simulink model "GeneralFramework"  (R2022a)
settings: Solver=ode23tb  StartTime=0.0  StopTime=t_sim  RelTol=1e-3
values from neighbouring files (symbols this model uses):
  AccPwrbp = [0 3.0779560993538198]    [Init_Parameters.m]
  AccSpdbp = [256.49641719585139 641.24104298962845]    [Init_Parameters.m]
  EngTrqSat = 60    [Init_Parameters.m]
  f_mu = ones(4,1)    [Init_Parameters.m]
  InitialLatPosition = 0    [Init_Parameters.m]
  numWheels = 4    [Init_Parameters.m]    (also in VehicleParameters.m)
  omega_hw = 13.51    [Init_Parameters.m]
  steerDir = -1    [Init_Parameters.m]
  t_start = 1    [Init_Parameters.m]
  t_stop = 100    [Init_Parameters.m]
  theta_max = 270    [Init_Parameters.m]
  TrackWidth = VEH.TrackWidth    [Init_Parameters.m]
  Trans = data.Trans    [Init_Parameters.m]    (also in ModelWorkspace.mat = )
  VEH = data.VEH    [Init_Parameters.m]    (also in ModelWorkspace.mat = ; VehicleParameters.m)
  wheelB = VEH.FrontAxlePositionfromCG+VEH.RearAxlePositionfromCG    [Init_Parameters.m]    (also in VehicleParameters.m)
  xdot_r = 2    [Init_Parameters.m]
libraries: autolibutils x10, simulink x8, sharedtransform x5, autolibsharedcoupling x3, vehdynlibsuspension x2, shared6dof x2, autolibtranscontrolscommon x1, vehdynlibdriver x1, autolibsharedtransfixedgear x1, vehdynlibsteering x1, autolibshareddiff x1, autolibsharedmappedengines x1
(part 3 of 5)

== system GeneralFramework/Passanger Vehicle/Pedal Cluster Input ==
  Driver : Inport
  Driveline : Inport  Port=2
  Steering : Inport  Port=3
  Bus Selector : BusSelector  OutputSignals=SteerCmd,AccelCmd,DecelCmd,GearCmd
  Bus Selector1 : BusSelector  OutputSignals=BrkPrs
  Bus Selector2 : BusSelector  OutputSignals=StrWhlTrq
  SteerCmd : Outport  VectorParamsAs1DForOutWhenUnconnected=off
  AccelCmd : Outport  Port=2  VectorParamsAs1DForOutWhenUnconnected=off
  DecelCmd : Outport  Port=3  VectorParamsAs1DForOutWhenUnconnected=off
  GearCmd : Outport  Port=4  VectorParamsAs1DForOutWhenUnconnected=off
  BrkPrs : Outport  Port=5  VectorParamsAs1DForOutWhenUnconnected=off
  StrWhlTrq : Outport  Port=6  VectorParamsAs1DForOutWhenUnconnected=off
  wires:
  Bus Selector/2 -> AccelCmd/1  "<AccelCmd>"
  Driver/1 -> Bus Selector/1
  Bus Selector/3 -> DecelCmd/1  "<DecelCmd>"
  Bus Selector/4 -> GearCmd/1  "<GearCmd>"
  Bus Selector/1 -> SteerCmd/1  "<SteerCmd>"
  Driveline/1 -> Bus Selector1/1
  Bus Selector1/1 -> BrkPrs/1  "<BrkPrs>"
  Steering/1 -> Bus Selector2/1
  Bus Selector2/1 -> StrWhlTrq/1  "<StrWhlTrq>"

== system GeneralFramework/Passanger Vehicle/Pedal Cluster Output ==
  SteerFdbk : Inport
  AccFdbk : Inport  Port=2
  DecelFdbk : Inport  Port=3
  GearFdbk : Inport  Port=4
  Bus Creator1 : BusCreator  Inputs=4
  Signal Specification : SignalSpecification  Unit=rad
  Signal Specification1 : SignalSpecification  Unit=1
  Signal Specification2 : SignalSpecification  Unit=1
  Signal Specification3 : SignalSpecification  Unit=1
  OperatorFdbk : Outport
  wires:
  Signal Specification1/1 -> Bus Creator1/2  "AccFdbk"
  Signal Specification3/1 -> Bus Creator1/4  "GearFdbk"
  AccFdbk/1 -> Signal Specification1/1
  DecelFdbk/1 -> Signal Specification2/1
  GearFdbk/1 -> Signal Specification3/1
  Signal Specification/1 -> Bus Creator1/1  "SteerFdbk"
  SteerFdbk/1 -> Signal Specification/1
  Bus Creator1/1 -> OperatorFdbk/1
  Signal Specification2/1 -> Bus Creator1/3  "DecelFdbk"

== system GeneralFramework/Passanger Vehicle/Pedal Cluster and cabin ==
  SteerCmd : Inport
  AccCmd : Inport  Port=2
  DecelCmd : Inport  Port=3
  GearCmd : Inport  Port=4
  BrkPrs : Inport  Port=5
  StrWhlTrq : Inport  Port=6
  Brake Pedal : Subsystem
  Dead Zone2 : DeadZone  LowerValue=0  UpperValue=.01  ZeroCross=off
  Dead Zone3 : DeadZone  LowerValue=-.01  UpperValue=.01  ZeroCross=off
  Terminator : Terminator
  Terminator1 : Terminator
  SteerFdbk : Outport
  AccFdbk : Outport  Port=2
  DecelFdbk : Outport  Port=3
  GearFdbk : Outport  Port=4
  wires:
  AccCmd/1 -> Dead Zone2/1
  GearCmd/1 -> GearFdbk/1
  Brake Pedal/1(DecelFdbk) -> DecelFdbk/1
  Dead Zone3/1 -> SteerFdbk/1
  StrWhlTrq/1 -> Terminator1/1
  DecelCmd/1 -> Brake Pedal/1(DecelCmd)
  SteerCmd/1 -> Dead Zone3/1
  BrkPrs/1 -> Terminator/1
  Dead Zone2/1 -> AccFdbk/1

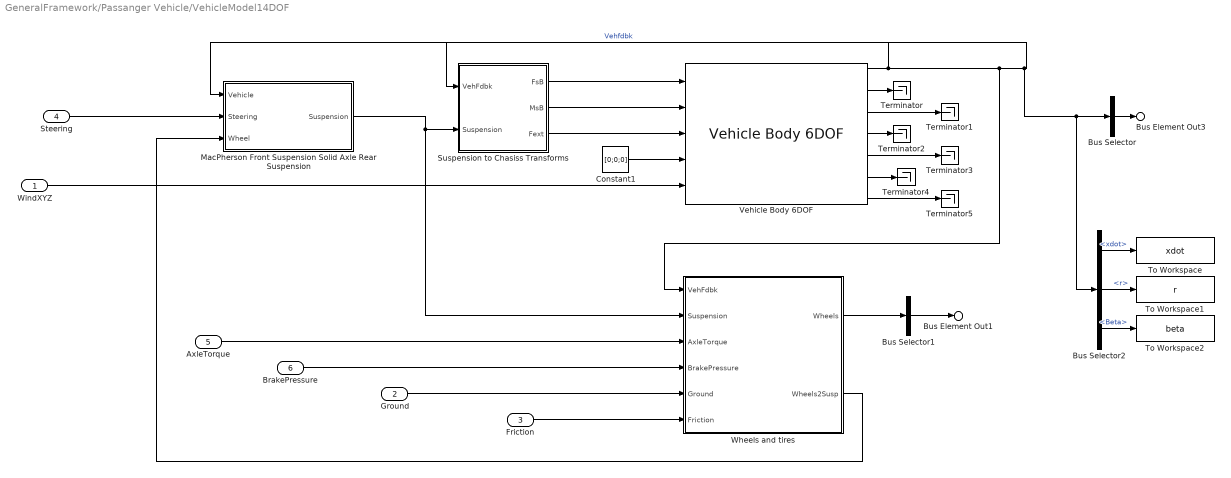
== system GeneralFramework/Passanger Vehicle/VehicleModel14DOF ==
  WindXYZ : Inport
  Ground : Inport  Port=2
  Friction : Inport  Port=3
  Steering : Inport  Port=4
  AxleTorque : Inport  Port=5
  BrakePressure : Inport  Port=6
  Bus Selector : BusSelector  OutputSignals=InertFrm,BdyFrm  OutputAsBus=on
  Bus Selector1 : BusSelector  OutputSignals=TireFrame,Steering  OutputAsBus=on
  Bus Selector2 : BusSelector  OutputSignals=BdyFrm.Cg.Vel.xdot,BdyFrm.Cg.AngVel.r,BdyFrm.Geom.Ang.Beta
  Constant1 : Constant  Value=[0;0;0]
  MacPherson Front Suspension Solid Axle Rear Suspension : Subsystem
  Suspension to Chasiss Transforms : Subsystem
  Terminator{,1..5} (6 alike) : Terminator
  To Workspace : ToWorkspace  VariableName=xdot  SampleTime=-1
      settings: Save2DSignal=2-D array (concatenate along first dimension)
  To Workspace1 : ToWorkspace  VariableName=r  SampleTime=-1
      settings: Save2DSignal=2-D array (concatenate along first dimension)
  To Workspace2 : ToWorkspace  VariableName=beta  SampleTime=-1
      settings: Save2DSignal=2-D array (concatenate along first dimension)
  Vehicle Body 6DOF : vehdynlibeom/Vehicle Body 6DOF  extPos=on  extVel=on  extEuler=on  extRotRate=on  htchFMode=off  htchMMode=off  m=VEH.Mass  a=VEH.FrontAxlePositionfromCG  b=VEH.RearAxlePositionfromCG  d=0  h=VEH.HeightCG  dh=1  hl=0  hh=0.1  Xe_o=[VEH.InitialLongPosition,InitialLatPosition,VEH.InitialVertPosition]  xbdot_o=[VEH.InitialLongVel,VEH.InitialLatVel,VEH.InitialVertVel]  eul_o=[VEH.InitialRollAngle,VEH.InitialPitchAngle,VEH.InitialYawAngle]  p_o=[VEH.InitialRollRate,VEH.InitialPitchRate,VEH.InitialYawRate]  Iveh=[VEH.RollMomentInertia 0 0; 0 VEH.PitchMomentInertia 0; 0 0 VEH.YawMomentInertia]  w=VEH.TrackWidth.*[1 1]  z1m=0  z1R=[-.25,.125,.15]  z1I=[1.4,-.2,.1;-.2,1.4,.1;.1,.1,2.25].*0  z2m=0  z2R=[1.4,0,.8]  z2I=[1.4,-.2,.1;-.2,1.4,.1;.1,.1,2.25].*0  z3m=0  z3R=[.75,-.5,.4]  z3I=[5,-.1,-2;-2,9,.1;-.1,.1,6].*0  z4m=0  z4R=[.75,.5,.4]  z4I=[5,-.1,-2;-2,9,.1;-.1,.1,6].*0  z5m=0  z5R=[1.25,-.5,.4]  z5I=[5,-.1,-2;-2,9,.1;-.1,.1,6].*0  z6m=0  z6R=[1.25,-.5,.4]  z6I=[5,-.1,-2;-2,9,.1;-.1,.1,6].*0  z7m=0  z7R=[2,0,.25]  z7I=[1.4,-.2,.1;-.2,1.4,.1;.1,.1,2.25].*0  Af=VEH.FrontalArea  Cd=.3  Cl=.1  Cpm=.1  beta_w=[0 0.01:0.01:0.3]  Cs=[0 0.01:0.01:0.3]  Cym=[0 1e-6:0.01:0.3]  Pabs=101325  extTamb=off  Tair=273  g=9.81  xdot_tol=.1  longOff=0  latOff=0  vertOff=0.0112  wrapAng=off  aMode=2
      settings: SourceProductBaseCode=VE
  Wheels and tires : Subsystem
  Bus Element Out3 : Outport  PortName=Vehfdbk
  Bus Element Out1 : Outport  Port=2  PortName=Wheels
  wires:
  Ground/1 -> Wheels and tires/5(Ground)
  MacPherson Front Suspension Solid Axle Rear Suspension/1(Suspension) -> Wheels and tires/2(Suspension), Suspension to Chasiss Transforms/2(Suspension)
  Vehicle Body 6DOF/3 -> Terminator1/1
  Suspension to Chasiss Transforms/3(Fext) -> Vehicle Body 6DOF/3
  Vehicle Body 6DOF/7 -> Terminator5/1
  BrakePressure/1 -> Wheels and tires/4(BrakePressure)
  AxleTorque/1 -> Wheels and tires/3(AxleTorque)
  Vehicle Body 6DOF/6 -> Terminator4/1
  Vehicle Body 6DOF/5 -> Terminator3/1
  Constant1/1 -> Vehicle Body 6DOF/4
  Wheels and tires/2(Wheels2Susp) -> MacPherson Front Suspension Solid Axle Rear Suspension/3(Wheel)
  Vehicle Body 6DOF/4 -> Terminator2/1
  Suspension to Chasiss Transforms/1(FsB) -> Vehicle Body 6DOF/1
  Vehicle Body 6DOF/2 -> Terminator/1
  Suspension to Chasiss Transforms/2(MsB) -> Vehicle Body 6DOF/2
  WindXYZ/1 -> Vehicle Body 6DOF/5
  Steering/1 -> MacPherson Front Suspension Solid Axle Rear Suspension/2(Steering)
  Friction/1 -> Wheels and tires/6(Friction)
  Wheels and tires/1(Wheels) -> Bus Selector1/1
  Bus Selector1/1 -> Bus Element Out1/1
  Bus Selector/1 -> Bus Element Out3/1
  Vehicle Body 6DOF/1 -> Wheels and tires/1(VehFdbk), Bus Selector/1, Bus Selector2/1, MacPherson Front Suspension Solid Axle Rear Suspension/1(Vehicle), Suspension to Chasiss Transforms/1(VehFdbk)  "Vehfdbk"
  Bus Selector2/1 -> To Workspace/1  "<xdot>"
  Bus Selector2/2 -> To Workspace1/1  "<r>"
  Bus Selector2/3 -> To Workspace2/1  "<Beta>"

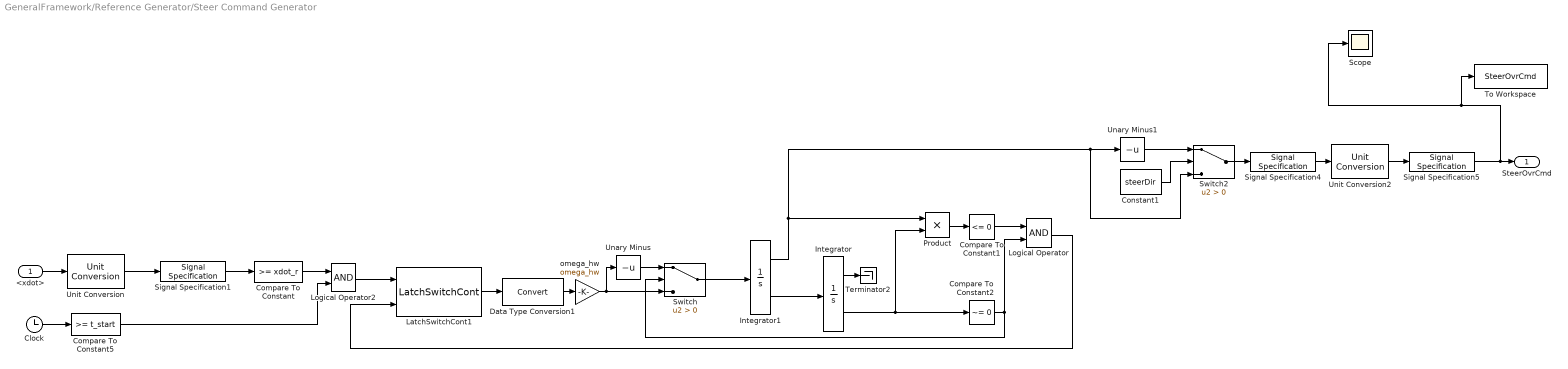
== system GeneralFramework/Reference Generator/Steer Command Generator ==
  <xdot> : Inport
  Clock : Clock
  Compare To Constant : simulink/Logic and Bit Operations/Compare To Constant  relop=>=  const=xdot_r  OutDataTypeStr=boolean
  Compare To Constant1 : simulink/Logic and Bit Operations/Compare To Constant  relop=<=  const=0  OutDataTypeStr=boolean
  Compare To Constant2 : simulink/Logic and Bit Operations/Compare To Constant  relop=~=  const=0  OutDataTypeStr=boolean  ZeroCross=off
  Compare To Constant5 : simulink/Logic and Bit Operations/Compare To Constant  relop=>=  const=t_start  OutDataTypeStr=boolean
  Constant1 : Constant  Value=steerDir
  Data Type Conversion1 : DataTypeConversion  SaturateOnIntegerOverflow=off  RndMeth=Floor
  Integrator : Integrator  LimitOutput=on  UpperSaturationLimit=t_stop  ShowSaturationPort=on
  Integrator1 : Integrator  LimitOutput=on  UpperSaturationLimit=theta_max  LowerSaturationLimit=-theta_max  ShowSaturationPort=on
  LatchSwitchCont1 : autolibutils/LatchSwitchCont  aMode=aMode
      settings: SourceProductBaseCode=PW,DR,MT,VE
  Logical Operator : Logic  AllPortsSameDT=off  OutDataTypeStr=boolean
  Logical Operator2 : Logic  AllPortsSameDT=off  OutDataTypeStr=boolean
  Product : Product
  Scope : Scope
  Signal Specification1 : SignalSpecification  Unit=mph
  Signal Specification4 : SignalSpecification  Unit=deg
  Signal Specification5 : SignalSpecification  Unit=rad
  Switch : Switch  Criteria=u2 > Threshold  SaturateOnIntegerOverflow=off  InputSameDT=off
  Switch2 : Switch  Criteria=u2 > Threshold  SaturateOnIntegerOverflow=off  InputSameDT=off
  Terminator2 : Terminator
  To Workspace : ToWorkspace  VariableName=SteerOvrCmd  SampleTime=-1
      settings: Save2DSignal=2-D array (concatenate along first dimension)
  Unary Minus : UnaryMinus
  Unary Minus1 : UnaryMinus
  Unit Conversion : UnitConversion
  Unit Conversion2 : UnitConversion
  omega_hw : Gain  Gain=omega_hw
  SteerOvrCmd : Outport  VectorParamsAs1DForOutWhenUnconnected=off
  wires:
  Unit Conversion2/1 -> Signal Specification5/1
  Unary Minus/1 -> Switch/1
  Compare To Constant/1 -> Logical Operator2/1
  Unary Minus1/1 -> Switch2/1
  Switch/1 -> Integrator1/1
  Signal Specification4/1 -> Unit Conversion2/1
  Integrator1/1 -> Product/1, Unary Minus1/1, Switch2/3
  omega_hw/1 -> Switch/3, Unary Minus/1
  Compare To Constant1/1 -> Logical Operator/1
  <xdot>/1 -> Unit Conversion/1
  Clock/1 -> Compare To Constant5/1
  Data Type Conversion1/1 -> omega_hw/1
  Product/1 -> Compare To Constant1/1
  Unit Conversion/1 -> Signal Specification1/1
  Integrator/2 -> Product/2, Compare To Constant2/1
  Switch2/1 -> Signal Specification4/1
  Integrator/1 -> Terminator2/1
  Compare To Constant5/1 -> Logical Operator2/2
  Compare To Constant2/1 -> Logical Operator/2, Switch/2
  Signal Specification1/1 -> Compare To Constant/1
  Logical Operator2/1 -> LatchSwitchCont1/1
  Integrator1/2 -> Integrator/1
  Logical Operator/1 -> LatchSwitchCont1/2
  Constant1/1 -> Switch2/2
  LatchSwitchCont1/1 -> Data Type Conversion1/1
  Signal Specification5/1 -> To Workspace/1, Scope/1, SteerOvrCmd/1

== system GeneralFramework/Visualization/3D Engine ==
  note: 1) Add Subsystem or Model blocks as valid variant choices.
      | 2) You cannot connect blocks at this level. At simulation, connectivity is automatically
      | determined, based on the active variant and port name matching.
  VehFdbk : Inport
  3D Engine : Subsystem  VariantControl=engine3D==1
  3D Engine Disabled : Subsystem  VariantControl=engine3D==2

== system GeneralFramework/Visualization/ISO 15037-1:2006 ==
  VehFdbk : Inport
  Disabled : Subsystem  VariantControl=0
  Enabled : Subsystem  VariantControl=1

== system GeneralFramework/Passanger Vehicle/Driveline Idea Fixed Gear/Brake Hydraulics ==
  BrkPrsCmd : Inport
  Circuit : Switch  Criteria=u2 ~= 0  SaturateOnIntegerOverflow=off  InputSameDT=off
  Constant : Constant  Value=-1
  Front Bias : Constant
  Gain4 : Gain  Gain=8e6
  Mux : Mux
  Product : Product
  Rear Bias : Constant  Value=.6
  Scope : Scope
  Spool : Gain  Gain=50
  Subtract : Sum  Inputs=+-
  Valve : autolibutils/Cont LPF  wc=20*2*pi  AbsoluteTolerance=auto  aMode=2
      settings: SourceProductBaseCode=PW,DR,MT,VE
  Volume : Integrator  LimitOutput=on  UpperSaturationLimit=1  LowerSaturationLimit=0
  BrkPrs : Outport  VectorParamsAs1DForOutWhenUnconnected=off
  wires:
  Volume/1 -> Subtract/2, Product/2
  Valve/1 -> Volume/1  "Flow"
  BrkPrsCmd/1 -> Circuit/1, Circuit/2
  Gain4/1 -> Scope/1, BrkPrs/1
  Circuit/1 -> Subtract/1
  Constant/1 -> Circuit/3
  Subtract/1 -> Spool/1
  Spool/1 -> Valve/1
  Front Bias/1 -> Mux/2, Mux/1
  Rear Bias/1 -> Mux/3, Mux/4
  Product/1 -> Gain4/1
  Mux/1 -> Product/1

== system GeneralFramework/Passanger Vehicle/Driveline Idea Fixed Gear/Idea Trasmission ==
  Gear : Inport
  EngTrq : Inport  Port=2
  CSpd : Inport  Port=3
  Ideal Fixed Gear Transmission : autolibsharedtransfixedgear/Ideal Fixed Gear Transmission  VariantControl=0  TransEffModelPopup=Gear only  gearInterp=Linear point-slope  G=Trans.GearNums  Trq_bpts=[25, 50, 75, 100, 150, 200, 250]  omega_bpts=[52.4 78.5 105 131 157 183 209 262 314 419 524]  Temp_bpts=[313 358]  N=Trans.GearRatios  Jout=Trans.Inertias  bout=Trans.DampingCoeffs  eta=Trans.Efficiencies  eta_tbl=reshape([0.53 0.71 0.77 0.79 0.82 0.82 0.82 0.5 0.7 0.77 0.79 0.82 0.82 0.82 0.54 0.72 0.78 0.81 0.83 0.82 0.82 0.56 0.73 0.79 0.81 0.84 0.82 0.82 0.58 0.74 0.79 0.82 0.84 0.82 0.82 0.57 0.74 0.79 0.82 0.84 0.82 0.82 0.58 0.74 0.79 0.82 0.84 0.82 0.82 0.58 0.74 0.79 0.82 0.84 0.82 0.82 0.57 0.74 0.8 0.82 0.85 0.82 0.82 0.55 0.73 0.78 0.81 0.84 0.82 0.82 0.51 0.71 0.77 0.81 0.84 0.82 0.82 0.53 0.71 0.77 0.79 0.82 0.82 0.82 0.5 0.7 0.77 0.79 0.82 0.82 0.82 0.54 0.72 0.78 0.81 0.83 0.82 0.82 0.56 0.73 0.79 0.81 0.84 0.82 0.82 0.58 0.74 0.79 0.82 0.84 0.82 0.82 0.57 0.74 0.79 0.82 0.84 0.82 0.82 0.58 0.74 0.79 0.82 0.84 0.82 0.82 0.58 0.74 0.79 0.82 0.84 0.82 0.82 0.57 0.74 0.8 0.82 0.85 0.82 0.82 0.55 0.73 0.78 0.81 0.84 0.82 0.82 0.51 0.71 0.77 0.81 0.84 0.82 0.82 0.53 0.71 0.77 0.79 0.82 0.82 0.82 0.5 0.7 0.77 0.79 0.82 0.82 0.82 0.54 0.72 0.78 0.81 0.83 0.82 0.82 0.56 0.73 0.79 0.81 0.84 0.82 0.82 0.58 0.74 0.79 0.82 0.84 0.82 0.82 0.57 0.74 0.79 0.82 0.84 0.82 0.82 0.58 0.74 0.79 0.82 0.84 0.82 0.82 0.58 0.74 0.79 0.82 0.84 0.82 0.82 0.57 0.74 0.8 0.82 0.85 0.82 0.82 0.55 0.73 0.78 0.81 0.84 0.82 0.82 0.51 0.71 0.77 0.81 0.84 0.82 0.82 0.7 0.79 0.82 0.83 0.84 0.84 0.84 0.63 0.76 0.8 0.82 0.83 0.84 0.84 0.58 0.74 0.79 0.81 0.83 0.84 0.84 0.58 0.74 0.79 0.81 0.83 0.84 0.84 0.58 0.74 0.79 0.81 0.84 0.84 0.84 0.57 0.73 0.78 0.81 0.84 0.85 0.84 0.57 0.73 0.79 0.81 0.84 0.85 0.84 0.56 0.73 0.78 0.81 0.83 0.85 0.84 0.55 0.73 0.78 0.81 0.84 0.85 0.84 0.52 0.71 0.77 0.8 0.83 0.85 0.84 0.48 0.69 0.76 0.79 0.83 0.84 0.84 0.64 0.76 0.8 0.81 0.83 0.84 0.84 0.56 0.73 0.78 0.8 0.83 0.84 0.84 0.54 0.71 0.77 0.8 0.82 0.84 0.84 0.53 0.71 0.77 0.8 0.83 0.84 0.84 0.51 0.71 0.77 0.8 0.83 0.84 0.85 0.52 0.7 0.77 0.8 0.83 0.84 0.85 0.51 0.71 0.76 0.79 0.83 0.84 0.85 0.5 0.69 0.76 0.79 0.82 0.84 0.85 0.45 0.68 0.75 0.78 0.82 0.84 0.85 0.43 0.67 0.74 0.78 0.81 0.83 0.84 0.38 0.63 0.71 0.75 0.8 0.82 0.83 0.65 0.79 0.84 0.85 0.88 0.89 0.89 0.56 0.75 0.81 0.83 0.86 0.88 0.89 0.52 0.72 0.79 0.83 0.86 0.88 0.88 0.51 0.72 0.79 0.83 0.86 0.88 0.89 0.49 0.71 0.78 0.82 0.86 0.88 0.89 0.47 0.7 0.78 0.82 0.86 0.87 0.88 0.45 0.69 0.77 0.81 0.85 0.87 0.88 0.4 0.67 0.75 0.8 0.84 0.86 0.88 0.3 0.64 0.73 0.78 0.83 0.86 0.87 0.17 0.55 0.67 0.73 0.8 0.83 0.85 0.089 0.45 0.61 0.69 0.77 0.81 0.83 0.61 0.75 0.82 0.84 0.87 0.87 0.88 0.54 0.73 0.8 0.82 0.86 0.87 0.88 0.51 0.71 0.79 0.82 0.86 0.87 0.88 0.52 0.72 0.79 0.82 0.86 0.87 0.89 0.52 0.72 0.8 0.83 0.86 0.88 0.89 0.53 0.72 0.79 0.82 0.86 0.87 0.89 0.5 0.7 0.78 0.82 0.86 0.88 0.88 0.46 0.69 0.77 0.81 0.85 0.87 0.88 0.4 0.67 0.75 0.8 0.83 0.86 0.88 0.33 0.64 0.73 0.78 0.83 0.85 0.87 0.33 0.64 0.73 0.78 0.83 0.85 0.87 0.78 0.85 0.87 0.88 0.89 0.89 0.89 0.73 0.83 0.86 0.88 0.89 0.89 0.89 0.72 0.83 0.86 0.88 0.89 0.89 0.89 0.72 0.83 0.87 0.89 0.9 0.89 0.89 0.72 0.83 0.87 0.88 0.9 0.89 0.89 0.71 0.83 0.87 0.88 0.9 0.89 0.89 0.71 0.83 0.86 0.88 0.9 0.89 0.89 0.7 0.82 0.86 0.88 0.9 0.89 0.89 0.69 0.82 0.86 0.88 0.9 0.89 0.89 0.67 0.81 0.86 0.88 0.9 0.89 0.89 0.63 0.79 0.85 0.87 0.89 0.89 0.89 0.78 0.85 0.87 0.88 0.89 0.89 0.89 0.73 0.83 0.86 0.88 0.89 0.89 0.89 0.72 0.83 0.86 0.88 0.89 0.89 0.89 0.72 0.83 0.87 0.89 0.9 0.89 0.89 0.72 0.83 0.87 0.88 0.9 0.89 0.89 0.71 0.83 0.87 0.88 0.9 0.89 0.89 0.71 0.83 0.86 0.88 0.9 0.89 0.89 0.7 0.82 0.86 0.88 0.9 0.89 0.89 0.69 0.82 0.86 0.88 0.9 0.89 0.89 0.67 0.81 0.86 0.88 0.9 0.89 0.89 0.63 0.79 0.85 0.87 0.89 0.89 0.89 0.78 0.85 0.87 0.88 0.89 0.89 0.89 0.73 0.83 0.86 0.88 0.89 0.89 0.89 0.72 0.83 0.86 0.88 0.89 0.89 0.89 0.72 0.83 0.87 0.89 0.9 0.89 0.89 0.72 0.83 0.87 0.88 0.9 0.89 0.89 0.71 0.83 0.87 0.88 0.9 0.89 0.89 0.71 0.83 0.86 0.88 0.9 0.89 0.89 0.7 0.82 0.86 0.88 0.9 0.89 0.89 0.69 0.82 0.86 0.88 0.9 0.89 0.89 0.67 0.81 0.86 0.88 0.9 0.89 0.89 0.63 0.79 0.85 0.87 0.89 0.89 0.89 0.82 0.87 0.88 0.89 0.89 0.89 0.89 0.81 0.87 0.89 0.89 0.9 0.9 0.89 0.76 0.85 0.87 0.89 0.9 0.89 0.89 0.72 0.83 0.86 0.88 0.89 0.89 0.89 0.72 0.83 0.86 0.88 0.89 0.9 0.89 0.71 0.82 0.86 0.88 0.89 0.9 ...(+1314 chars))  G_o=0  omega_o=0  omegaN_o=0  tau_s=Trans.ShiftTau  maxAbsSpd=5e3  aMode=2
      settings: SourceProductBaseCode=PW,DR,MT,VE
  One-way clutch : Saturate  UpperLimit=inf  LowerLimit=0
  Prop Shaft : autolibsharedcoupling/Torsional Compliance  port_config=Simulink  extInfo=off  k=5e3  b=10  theta_o=0  domega_o=0  omega_c=100  blkID=0  aMode=2
      settings: SourceProductBaseCode=PW,DR,MT,VE
  Scope : Scope
  Info : Outport
  EngSpd : Outport  Port=2
  CTrq : Outport  Port=3
  wires:
  Gear/1 -> Ideal Fixed Gear Transmission/1
  Prop Shaft/2 -> CTrq/1
  Ideal Fixed Gear Transmission/1 -> Info/1
  Prop Shaft/1 -> Ideal Fixed Gear Transmission/3
  Ideal Fixed Gear Transmission/3 -> Prop Shaft/1
  EngTrq/1 -> One-way clutch/1
  CSpd/1 -> Prop Shaft/2
  One-way clutch/1 -> Ideal Fixed Gear Transmission/2
  Ideal Fixed Gear Transmission/2 -> Scope/1, EngSpd/1

== system GeneralFramework/Passanger Vehicle/Driveline Idea Fixed Gear/Kinemartic stee ==
  AngIn : Inport
  Ground : Ground
  Ground3 : Ground
  Kinematic Steering : vehdynlibsteering/Kinematic Steering  StrgType=Ackerman  StrgRatioType=Constant  Loc=Front  NrmlFctr=1  TrckWdth=1.922  WhlBase=(1.515+1.504)  Db=0  StrgRng=3*pi  StrgAngBpts="[-6.2832   -5.0265   -3.7699   -2.5133   -1.2566         0    1.2566    2.5133    3.7699    5.0265    6.2832]"  StrgRatioTbl=|  StrgRatio=18  PctAckIn=off  PctAck=100  PctAckTbl=ones(1,11)*100  StrgArmLngth=0.1  RckCsLngth=0.5  TieRodLngth=0.248128028933392  D=0.2  PnnRadius=0.0057  PnnRadiusTbl="[0.0055    0.0055    0.0056    0.0057    0.0057    0.0057    0.0057    0.0057    0.0056    0.0055    0.0055]"  RodLngth=0.1  ParaArmLngth=0.9  aMode=2
      | [13.5000   13.3750   13.2500   13.1250   13.0000   13.0000   13.0000   13.1250   13.2500   13.3750   13.5000
      | ]
  Terminator : Terminator
  Vector Concatenate : Concatenate
  Vector Concatenate1 : Concatenate
  Vector Concatenate2 : Concatenate
  WhlAng : Outport
  StrWhlTrq : Outport  Port=2
  wires:
  Vector Concatenate2/1 -> Vector Concatenate1/2  "RearWheelAngles"
  Vector Concatenate/1 -> Vector Concatenate1/1  "FrontWheelAngles"
  Kinematic Steering/2 -> Vector Concatenate/1
  Ground3/1 -> Vector Concatenate2/2, Vector Concatenate2/1
  Vector Concatenate1/1 -> WhlAng/1
  Kinematic Steering/3 -> Vector Concatenate/2
  AngIn/1 -> Kinematic Steering/1
  Kinematic Steering/1 -> Terminator/1
  Ground/1 -> StrWhlTrq/1

== system GeneralFramework/Passanger Vehicle/Driveline Idea Fixed Gear/Rear wheel Active differential ==
  DriveshftTrq : Inport
  Omega : Inport  Port=2
  DiffPrsCmd : Inport  Port=3
  Active Differential : autolibshareddiff/Active Differential  diffType=Spur gears, superposition clutches  Ns1=.875  Ns2=1.125  Jgc=.003  Np1=1.125  Js1=.001  Jc1=.001  Jr1=.002  Np2=1.125  Js2=.001  Jc2=0.001  Jr2=0.002  shaftSwitchMask=To the left of center-line  Ndiff=Trans.FinalDrive  Jd=.08  bd=1e-3  Jw1=.01  bw1=1e-3  Jw2=.01  bw2=1e-3  omegaw1o=0  omegaw2o=0  couplingType=Pre-loaded ideal clutch  Aeff=0.01  Ndisks=4  Reff=.08  Fc=0  muc=[.16 0.13 0.115 0.11 0.105 0.1025 0.10125 .10125]  dw=[0 10 20 40 60 80 100 1000]  TdPdw=[-1000, -500, -90, -50, -5, 0, 5, 50, 90, 500, 1000].*ones(11)  pT=[0 1e3 5e3 7e3 1e4 2e4 5e4 1e5 5e5 1e6 5e6]  dwT=[-500 -200, -175, -100, - 50, 0, 50, 100, 175, 200, 500]  tauC=.04  IdealInterpMethod=Linear point-slope  IdealExtrapMethod=Clip  TdwInterpMethod=Linear point-slope  TdwExtrapMethod=Clip  maxAbsSpd=5e3  aMode=2  blkID=0
      settings: SourceProductBaseCode=PW,DR,MT,VE
  Demux : Demux  Outputs=[2,2]
  Demux1 : Demux  Outputs=2
  Demux2 : Demux  Outputs=2
  Ground : Ground
  Ground1 : Ground
  Scope : Scope
  Selector : Selector  InputPortWidth=4  IndexOptions=Index vector (dialog)  Indices=[3 4]  OutputSizes=1
  Terminator : Terminator
  Terminator1 : Terminator
  Torsional Compliance : autolibsharedcoupling/Torsional Compliance  port_config=Simulink  extInfo=off  k=5e3  b=10  theta_o=0  domega_o=0  omega_c=100  blkID=0  aMode=2
      settings: SourceProductBaseCode=PW,DR,MT,VE
  Torsional Compliance1 : autolibsharedcoupling/Torsional Compliance  port_config=Simulink  extInfo=off  k=5e3  b=10  theta_o=0  domega_o=0  omega_c=100  blkID=0  aMode=2
      settings: SourceProductBaseCode=PW,DR,MT,VE
  Vector Concatenate : Concatenate  NumInputs=4
  PromptShaftSpd : Outport
  DriveshftSpd : Outport  Port=2
  wires:
  Selector/1 -> Demux2/1
  Demux/2 -> Demux1/1
  Active Differential/1 -> Terminator/1
  Torsional Compliance/2 -> Vector Concatenate/3
  Torsional Compliance1/2 -> Scope/1, Vector Concatenate/4
  Demux2/2 -> Active Differential/2
  Demux2/1 -> Active Differential/1
  Demux1/2 -> Torsional Compliance1/2
  Demux1/1 -> Torsional Compliance/2
  Torsional Compliance1/1 -> Active Differential/5
  Demux/1 -> Terminator1/1
  Active Differential/3 -> Torsional Compliance/1
  DriveshftTrq/1 -> Active Differential/3
  Torsional Compliance/1 -> Active Differential/4
  Ground/1 -> Vector Concatenate/2
  Omega/1 -> Demux/1
  Active Differential/4 -> Torsional Compliance1/1
  Ground1/1 -> Vector Concatenate/1
  Vector Concatenate/1 -> PromptShaftSpd/1
  DiffPrsCmd/1 -> Selector/1
  Active Differential/2 -> DriveshftSpd/1

== system GeneralFramework/Passanger Vehicle/Idela Mapped Engine/Accessory Load Model ==
  EngTrqIn : Inport
  EngSpd : Inport  Port=2
  Accessory Load Power : Lookup_n-D  NumberOfTableDimensions=1  LookupTableObject=''  BreakpointsForDimension1=AccSpdbp  Table=AccPwrbp  ExtrapMethod=Clip  InternalRulePriority=Speed  RndMeth=Simplest
  Divide : Product  Inputs=*/
  Kw to w : Gain  Gain=1000
  Net Torque : Sum  Inputs=+-
  Saturation : Saturate  UpperLimit=Inf  LowerLimit=300
  rpm to rad/s : Gain  Gain=pi/30
  EngTrqOut : Outport  Unit=N*m  VectorParamsAs1DForOutWhenUnconnected=off
  wires:
  Divide/1 -> Net Torque/2
  Accessory Load Power/1 -> Kw to w/1
  EngSpd/1 -> Saturation/1, Accessory Load Power/1
  Saturation/1 -> rpm to rad/s/1
  rpm to rad/s/1 -> Divide/2
  Net Torque/1 -> EngTrqOut/1
  Kw to w/1 -> Divide/1
  EngTrqIn/1 -> Net Torque/1

== system GeneralFramework/Passanger Vehicle/Pedal Cluster and cabin/Brake Pedal ==
  DecelCmd : Inport
  Constant1 : Constant  Value=-20
  Dead Zone1 : DeadZone  LowerValue=0  UpperValue=.01  ZeroCross=off
  Gain3 : Gain
  Integrator2 : Integrator  LimitOutput=on  UpperSaturationLimit=1  LowerSaturationLimit=0
  Switch1 : Switch  Criteria=u2 > Threshold  Threshold=.1  SaturateOnIntegerOverflow=off  InputSameDT=off
  DecelFdbk : Outport
  wires:
  Dead Zone1/1 -> Switch1/2, Gain3/1
  Constant1/1 -> Switch1/3
  Integrator2/1 -> DecelFdbk/1
  Gain3/1 -> Switch1/1
  Switch1/1 -> Integrator2/1
  DecelCmd/1 -> Dead Zone1/1

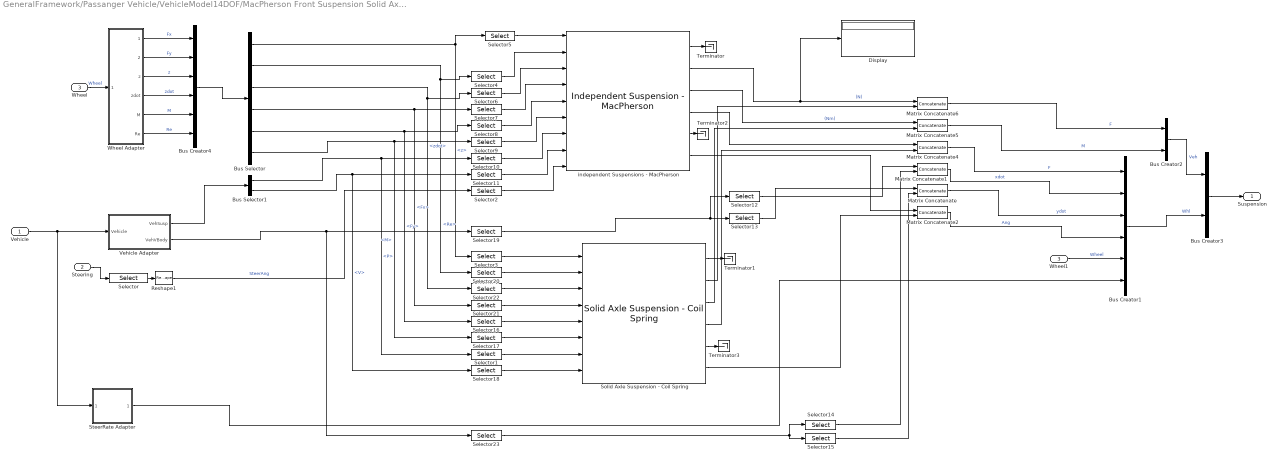
== system GeneralFramework/Passanger Vehicle/VehicleModel14DOF/MacPherson Front Suspension Solid Axle Rear Suspension ==
  Vehicle : Inport
  Steering : Inport  Port=2
  Wheel : Inport  Port=3
  Bus Creator1 : BusCreator  Inputs=6
  Bus Creator2 : BusCreator  Inputs=2
  Bus Creator3 : BusCreator  Inputs=2
  Bus Creator4 : BusCreator  Inputs=6
  Bus Selector : BusSelector  OutputSignals=z,Re,zdot,Fx,Fy,M
  Bus Selector1 : BusSelector  OutputSignals=P,V
  Display : Display
  Matrix Concatenate{,1..2,4..6} (6 alike) : Concatenate  Mode=Multidimensional array  ConcatenateDimension=2
  Reshape1 : Reshape  OutputDimensionality=Row vector (2-D)
  Selector{,2,4..8} (7 alike) : Selector  IndexOptions=Index vector (dialog)  Indices=[1 2]  OutputSizes=1
  Selector{1,17..18,23} (4 alike) : Selector  NumberOfDimensions=2  IndexOptions=Select all,Index vector (dialog)  Indices=[1 2],[3 4]  OutputSizes=1,1
  Selector{9..11,19} (4 alike) : Selector  NumberOfDimensions=2  IndexOptions=Select all,Index vector (dialog)  Indices=[1 2],[1 2]  OutputSizes=1,1
  Selector12 : Selector  NumberOfDimensions=2  InputPortWidth=3  IndexOptions=Index vector (dialog),Select all  Indices=1,1  OutputSizes=1,1
  Selector13 : Selector  NumberOfDimensions=2  InputPortWidth=3  IndexOptions=Index vector (dialog),Select all  Indices=2,1  OutputSizes=1,1
  Selector14 : Selector  NumberOfDimensions=2  InputPortWidth=3  IndexOptions=Index vector (dialog),Select all  Indices=1,1  OutputSizes=1,1
  Selector15 : Selector  NumberOfDimensions=2  InputPortWidth=3  IndexOptions=Index vector (dialog),Select all  Indices=2,1  OutputSizes=1,1
  Selector{3,16,20..22} (5 alike) : Selector  IndexOptions=Index vector (dialog)  Indices=[3 4]  OutputSizes=1
  Solid Axle Suspension - Coil Spring : vehdynlibsuspension/Solid Axle Suspension - Coil Spring  NumAxl=1  NumTracksByAxl=2  StrgEnByAxl=0  TrackNumVec="[1  2]"  AxleNumVec="[1  1]"  SuspTypesByAxle=[1]  SuspImage=suspsacoil.png  AxlIxx=AxlIxx  AxlM=AxlM  TrackCoords=[0 0;VEH.TrackWidth*[-1 1]/2;0 0]  SuspCoords=[0 0;VEH.TrackWidth*[-1 1]/2;0 0]  KzWhlAxl=KzWhlAxl  F0zWhlAxl=F0zWhlAxl  CzWhlAxl=CzWhlAxl  IdealSuspEn=on  IdealSuspAxles=[1]  Kz=Kz  F0z=F0zCS  Cz=Cz  Hmax=Hmax  Toe=0.  RollStrgSlp=0.  ToeStrgSlp=0  Caster=0.  CasterHslp=0.  CasterStrgSlp=0.01  Camber=0.  CamberHslp=0.  CamberStrgSlp=0.01  StrgHgtSlp=0.1432  MappedSuspEn=off  MappedSuspAxles="[1  2]"  f_susp_axl_bp=[1 2]  f_susp_dz_bp=[-0.15 -0.14 -0.13 -0.12 -0.11 -0.10 -0.09 -0.08 -0.07 -0.06 -0.05 -0.04 -0.03 -0.02 -0.01 0.00 0.01 0.02 0.03 0.04 0.05 0.06 0.07 0.08 0.09 0.10 0.11 0.12 0.13 0.14 0.15]  f_susp_dzdot_bp=[-0.15 -0.14 -0.13 -0.12 -0.11 -0.10 -0.09 -0.08 -0.07 -0.06 -0.05 -0.04 -0.03 -0.02 -0.01 0.00 0.01 0.02 0.03 0.04 0.05 0.06 0.07 0.08 0.09 0.10 0.11 0.12 0.13 0.14 0.15]  f_susp_fmz=zeros(31,31,61,2,4)  f_susp_geom=zeros(31,61,2,3)  f_susp_strgdelta_bp=[-30,-29,-28,-27,-26,-25,-24,-23,-22,-21,-20,-19,-18,-17,-16,-15,-14,-13,-12,-11,-10,-9,-8,-7,-6,-5,-4,-3,-2,-1,0,1,2,3,4,5,6,7,8,9,10,11,12,13,14,15,16,17,18,19,20,21,22,23,24,25,26,27,28,29,30]
      settings: SourceProductBaseCode=VE
  SteerRate Adapter : Subsystem
  Terminator{,1..3} (4 alike) : Terminator
  Vehicle Adapter : Subsystem
  Wheel Adapter : Subsystem
  Wheel1 : InportShadow  Port=3
  independent Suspensions - MacPherson : vehdynlibsuspension/Independent Suspension - MacPherson  ActiveDampEn=off  NumAxl=1  NumTracksByAxl=2  StrgEnByAxl=1  AntiSwayEnByAxl=1  TrackNumVec="[1  2]"  AxleNumVec="[1  1]"  SuspTypesByAxle=[1]  SuspImage=suspmacp.png  IdealSuspEn=on  IdealSuspAxles=[1]  Kz=Kz  F0z=F0zMP  Cz=Cz  Hmax=Hmax  f_act_susp_cz=[10000 10000;10000 10000]  f_act_susp_duty_bpt=[0 1]  f_act_susp_zdot_bpt=[-1 1]  Toe=0  RollStrgSlp=0.  ToeStrgSlp=0.  Caster=0.  CasterHslp=0.  CasterStrgSlp=0.  Camber=-0.5*pi/180*0  CamberHslp=0.  CamberStrgSlp=0.  StrgHgtSlp=0.1432  MappedSuspEn=off  MappedSuspAxles="[1  2]"  f_susp_axl_bp=[1 2]  f_susp_dz_bp=[-0.15 -0.14 -0.13 -0.12 -0.11 -0.10 -0.09 -0.08 -0.07 -0.06 -0.05 -0.04 -0.03 -0.02 -0.01 0.00 0.01 0.02 0.03 0.04 0.05 0.06 0.07 0.08 0.09 0.10 0.11 0.12 0.13 0.14 0.15]  f_susp_dzdot_bp=[-0.15 -0.14 -0.13 -0.12 -0.11 -0.10 -0.09 -0.08 -0.07 -0.06 -0.05 -0.04 -0.03 -0.02 -0.01 0.00 0.01 0.02 0.03 0.04 0.05 0.06 0.07 0.08 0.09 0.10 0.11 0.12 0.13 0.14 0.15]  f_susp_fmz=zeros(31,31,61,2,4)  f_susp_geom=zeros(31,61,2,3)  f_susp_strgdelta_bp=[-30,-29,-28,-27,-26,-25,-24,-23,-22,-21,-20,-19,-18,-17,-16,-15,-14,-13,-12,-11,-10,-9,-8,-7,-6,-5,-4,-3,-2,-1,0,1,2,3,4,5,6,7,8,9,10,11,12,13,14,15,16,17,18,19,20,21,22,23,24,25,26,27,28,29,30]  AntiSwayR=0.2  AntiSwayNtrlAng=0.5236  AntiSwayTrsK=8e+02
      settings: SourceProductBaseCode=VE
  Suspension : Outport  VectorParamsAs1DForOutWhenUnconnected=off
  wires:
  Wheel1/1 -> Bus Creator1/5  "Wheel"
  Bus Selector/5 -> Selector16/1, Selector8/1  "<Fy>"
  Vehicle Adapter/2(VehVBody) -> Selector23/1, Selector19/1
  Matrix Concatenate1/1 -> Bus Creator1/2  "xdot"
  Selector19/1 -> Selector12/1, Selector13/1
  Selector2/1 -> independent Suspensions - MacPherson/9
  Wheel Adapter/2(WhFy) -> Bus Creator4/2  "Fy"
  Selector11/1 -> independent Suspensions - MacPherson/8
  Bus Creator4/1 -> Bus Selector/1
  Bus Selector/2 -> Selector20/1, Selector4/1  "<Re>"
  Bus Selector1/2 -> Selector18/1, Selector11/1  "<V>"
  Solid Axle Suspension - Coil Spring/3 -> Matrix Concatenate5/2
  Vehicle/1 -> SteerRate Adapter/1(Vehicle), Vehicle Adapter/1(Vehicle)
  Solid Axle Suspension - Coil Spring/6 -> Matrix Concatenate2/2
  Solid Axle Suspension - Coil Spring/1 -> Terminator1/1
  Matrix Concatenate/1 -> Bus Creator1/3  "ydot"
  independent Suspensions - MacPherson/1 -> Terminator/1
  Wheel Adapter/5(M) -> Bus Creator4/5  "M"
  Selector10/1 -> independent Suspensions - MacPherson/7
  Selector23/1 -> Selector15/1, Selector14/1
  Wheel/1 -> Wheel Adapter/1(Wheels)  "Wheel"
  Wheel Adapter/4(zdot) -> Bus Creator4/4  "zdot"
  Selector17/1 -> Solid Axle Suspension - Coil Spring/6
  Wheel Adapter/1(WhFx) -> Bus Creator4/1  "Fx"
  Selector20/1 -> Solid Axle Suspension - Coil Spring/2
  Selector6/1 -> independent Suspensions - MacPherson/3
  Selector15/1 -> Matrix Concatenate/2
  Steering/1 -> Selector/1
  Selector18/1 -> Solid Axle Suspension - Coil Spring/8
  Selector16/1 -> Solid Axle Suspension - Coil Spring/5
  Selector7/1 -> independent Suspensions - MacPherson/4
  Matrix Concatenate4/1 -> Bus Creator1/1  "F"
  Solid Axle Suspension - Coil Spring/4 -> Matrix Concatenate4/2
  Selector8/1 -> independent Suspensions - MacPherson/5
  independent Suspensions - MacPherson/2 -> Display/1, Matrix Concatenate6/1  "(N)"
  Selector5/1 -> independent Suspensions - MacPherson/1
  Selector9/1 -> independent Suspensions - MacPherson/6
  Selector21/1 -> Solid Axle Suspension - Coil Spring/4
  Bus Selector1/1 -> Selector1/1, Selector10/1  "<P>"
  Selector3/1 -> Solid Axle Suspension - Coil Spring/1
  Solid Axle Suspension - Coil Spring/5 -> Terminator3/1
  Selector/1 -> Reshape1/1
  Bus Creator2/1 -> Bus Creator3/1  "Veh"
  Wheel Adapter/3(z) -> Bus Creator4/3  "z"
  Bus Selector/3 -> Selector22/1, Selector6/1  "<zdot>"
  Wheel Adapter/6(Re) -> Bus Creator4/6  "Re"
  Selector22/1 -> Solid Axle Suspension - Coil Spring/3
  Matrix Concatenate5/1 -> Bus Creator2/2  "M"
  independent Suspensions - MacPherson/4 -> Matrix Concatenate4/1
  Selector4/1 -> independent Suspensions - MacPherson/2
  Selector1/1 -> Solid Axle Suspension - Coil Spring/7
  Bus Selector/1 -> Selector3/1, Selector5/1  "<z>"
  Bus Selector/6 -> Selector17/1, Selector9/1  "<M>"
  Matrix Concatenate6/1 -> Bus Creator2/1  "F"
  Bus Creator3/1 -> Suspension/1
  Bus Selector/4 -> Selector21/1, Selector7/1  "<Fx>"
  Reshape1/1 -> Selector2/1  "SteerAng"
  independent Suspensions - MacPherson/5 -> Terminator2/1
  Vehicle Adapter/1(VehSusp) -> Bus Selector1/1
  Bus Creator1/1 -> Bus Creator3/2  "Whl"
  independent Suspensions - MacPherson/3 -> Matrix Concatenate5/1  "(Nm)"
  Selector12/1 -> Matrix Concatenate1/1
  Matrix Concatenate2/1 -> Bus Creator1/4  "Ang"
  Solid Axle Suspension - Coil Spring/2 -> Matrix Concatenate6/2
  Selector14/1 -> Matrix Concatenate1/2
  independent Suspensions - MacPherson/6 -> Matrix Concatenate2/1
  Selector13/1 -> Matrix Concatenate/1
  SteerRate Adapter/1(AngVel) -> Bus Creator1/6

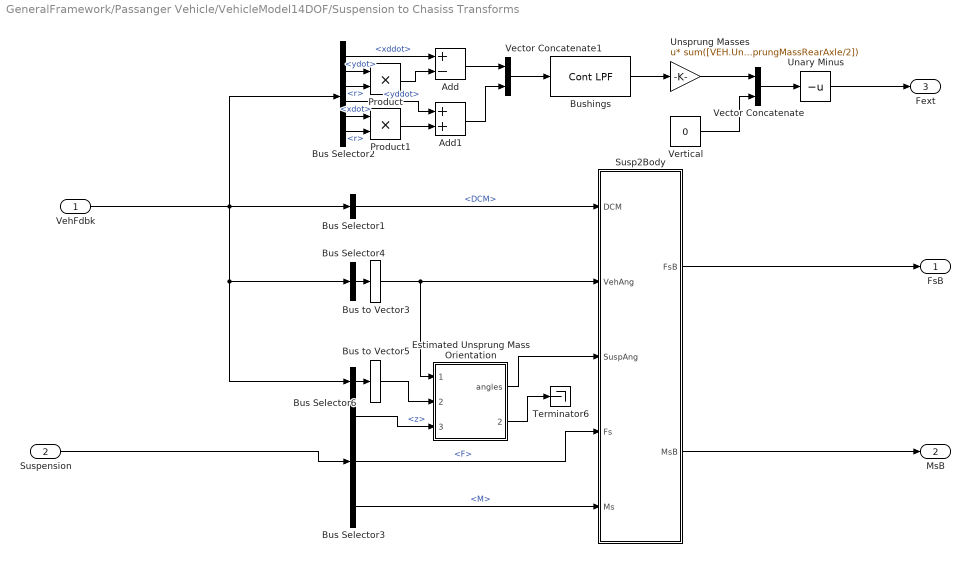
== system GeneralFramework/Passanger Vehicle/VehicleModel14DOF/Suspension to Chasiss Transforms ==
  VehFdbk : Inport
  Suspension : Inport  Port=2
  Add : Sum  Inputs=+-
  Add1 : Sum
  Bus Selector1 : BusSelector  OutputSignals=BdyFrm.Cg.DCM
  Bus Selector2 : BusSelector  OutputSignals=BdyFrm.Cg.Acc.xddot,BdyFrm.Cg.Vel.ydot,BdyFrm.Cg.AngVel.r,BdyFrm.Cg.Acc.yddot,BdyFrm.Cg.Vel.xdot,BdyFrm.Cg.AngVel.r
  Bus Selector3 : BusSelector  OutputSignals=Whl.Wheel.SuspFrame.z,Veh.F,Veh.M
  Bus Selector4 : BusSelector  OutputSignals=InertFrm.Cg.Ang.phi,InertFrm.Cg.Ang.theta,InertFrm.Cg.Ang.psi  OutputAsBus=on
  Bus Selector6 : BusSelector  OutputSignals=InertFrm.Geom.Disp.X,InertFrm.Geom.Disp.Y,InertFrm.Geom.Disp.Z  OutputAsBus=on
  Bus to Vector3 : BusToVector
  Bus to Vector5 : BusToVector
  Bushings : autolibutils/Cont LPF  wc=40*pi  AbsoluteTolerance=auto  aMode=2
      settings: SourceProductBaseCode=PW,DR,MT,VE
  Estimated Unsprung Mass Orientation : MATLAB Function  TreatAsAtomicUnit=on
  Product : Product
  Product1 : Product
  Susp2Body : Subsystem
  Terminator6 : Terminator
  Unary Minus : UnaryMinus
  Unsprung Masses : Gain  Gain=sum([VEH.UnsprungMassFrontAxle/2 VEH.UnsprungMassFrontAxle/2 VEH.UnsprungMassRearAxle/2 VEH.UnsprungMassRearAxle/2])  Multiplication=Matrix(u*K)
  Vector Concatenate : Concatenate
  Vector Concatenate1 : Concatenate
  Vertical : Constant  Value=0
  FsB : Outport
  MsB : Outport  Port=2
  Fext : Outport  Port=3
  wires:
  Estimated Unsprung Mass Orientation/1(angles) -> Susp2Body/3(SuspAng)
  Bus Selector3/1 -> Estimated Unsprung Mass Orientation/3(Ground)  "<z>"
  Vector Concatenate1/1 -> Bushings/1
  Bus Selector2/6 -> Product1/2  "<r>"
  Product/1 -> Add/2
  Bus Selector2/3 -> Product/2  "<r>"
  Bus Selector2/5 -> Product1/1  "<xdot>"
  Vertical/1 -> Vector Concatenate/2
  Add1/1 -> Vector Concatenate1/2
  Suspension/1 -> Bus Selector3/1
  Bushings/1 -> Unsprung Masses/1
  Vector Concatenate/1 -> Unary Minus/1
  VehFdbk/1 -> Bus Selector6/1, Bus Selector4/1, Bus Selector2/1, Bus Selector1/1
  Product1/1 -> Add1/2
  Bus to Vector3/1 -> Estimated Unsprung Mass Orientation/1(angleIn), Susp2Body/2(VehAng)
  Bus to Vector5/1 -> Estimated Unsprung Mass Orientation/2(GemoXYZIn)
  Unary Minus/1 -> Fext/1
  Bus Selector2/1 -> Add/1  "<xddot>"
  Add/1 -> Vector Concatenate1/1
  Bus Selector3/3 -> Susp2Body/5(Ms)  "<M>"
  Bus Selector2/2 -> Product/1  "<ydot>"
  Unsprung Masses/1 -> Vector Concatenate/1
  Estimated Unsprung Mass Orientation/2(GeomXYZ) -> Terminator6/1
  Bus Selector2/4 -> Add1/1  "<yddot>"
  Bus Selector3/2 -> Susp2Body/4(Fs)  "<F>"
  Bus Selector1/1 -> Susp2Body/1(DCM)  "<DCM>"
  Bus Selector6/1 -> Bus to Vector5/1
  Bus Selector4/1 -> Bus to Vector3/1
  Susp2Body/1(FsB) -> FsB/1
  Susp2Body/2(MsB) -> MsB/1
